simulink model "TESAOffense13"  (R2025b)
settings: Solver=FixedStepAuto  StartTime=0.0  StopTime=SimulationTime  FixedStep=timestep  RelTol=1e-3
values from neighbouring files (symbols this model uses):
  g = 9.81    [TESA_Workspace1.m]
  I = eye(3,3)    [TESA_Workspace1.m]
  K = [1 1 1 1 ... (first row only)    [TESA_Workspace1.m]
  m = 4.34    [TESA_Workspace1.m]    (also in min_snap_Coef.m = length(timepoints) - 1)
settings Model: Creator=worap  LastModifiedBy=btxs
settings DataIOCC: ExternalInput=inputStructure  LoadExternalInput=on

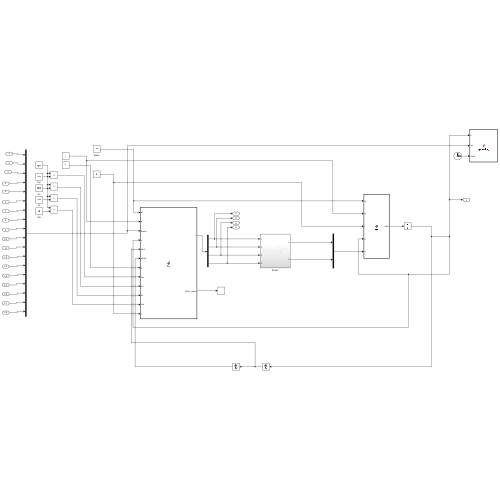
[thumbnail: Simulink's stored preview of the top-level diagram]
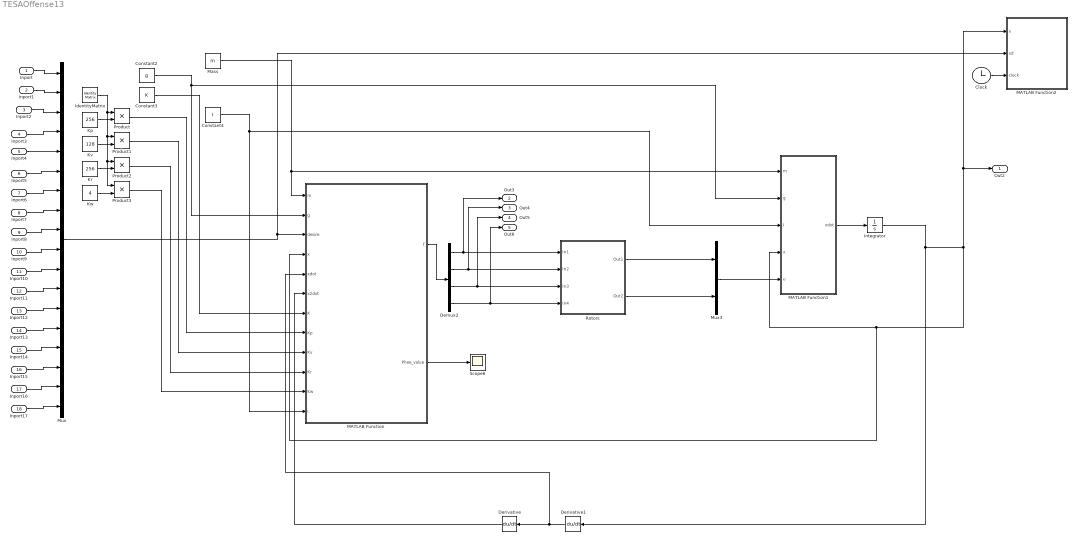
== system TESAOffense13 ==
  Inport : Inport
  Inport1 : Inport  Port=2
  Inport2 : Inport  Port=3
  Inport3 : Inport  Port=4
  Inport4 : Inport  Port=5
  Inport5 : Inport  Port=6
  Inport6 : Inport  Port=7
  Inport7 : Inport  Port=8
  Inport8 : Inport  Port=9
  Inport9 : Inport  Port=10
  Inport10 : Inport  Port=11
  Inport11 : Inport  Port=12
  Inport12 : Inport  Port=13
  Inport13 : Inport  Port=14
  Inport14 : Inport  Port=15
  Inport15 : Inport  Port=16
  Inport16 : Inport  Port=17
  Inport17 : Inport  Port=18
  Clock : Clock
  Constant2 : Constant  Value=g
  Constant3 : Constant  Value=K
  Constant4 : Constant  Value=I
  Demux2 : Demux
  Derivative : Derivative
  Derivative1 : Derivative
  IdentityMatrix : IdentityMatrix  OutputDimensions=3
  Integrator : Integrator  InitialCondition=[0;0;0;0;0;0;1;0;0;0;1;0;0;0;1;0;0;0]
  Kp : Constant  Value=256
  Kr : Constant  Value=256
  Kv : Constant  Value=128
  Kw : Constant  Value=4
  MATLAB Function : MATLAB Function  TreatAsAtomicUnit=on
  MATLAB Function1 : MATLAB Function  TreatAsAtomicUnit=on
  MATLAB Function2 : MATLAB Function  TreatAsAtomicUnit=on
  Mass : Constant  Value=m
  Mux : Mux  Inputs=18
  Mux3 : Mux  Inputs=2
  Product{,1..3} (4 alike) : Product
  Rotors : Subsystem
  Scope6 : Scope
      settings: ActiveDisplayYMinimum=-0.44275151158705367  ActiveDisplayYMaximum=-0.10480685049587157
  Out2 : Outport
  Out3 : Outport  Port=2
  Out4 : Outport  Port=3
  Out5 : Outport  Port=4
  Out6 : Outport  Port=5
  wires:
  Mass/1 -> MATLAB Function1/1(m), MATLAB Function/1(m)
  Demux2/2 -> Out4/1, Rotors/2(In2)
  Rotors/1(Out1) -> Mux3/1
  Rotors/2(Out2) -> Mux3/2
  Demux2/3 -> Out5/1, Rotors/3(In3)
  Demux2/4 -> Out6/1, Rotors/4(In4)
  Constant4/1 -> MATLAB Function1/3(I), MATLAB Function/12(I)
  MATLAB Function/1(f) -> Demux2/1
  Demux2/1 -> Out3/1, Rotors/1(In1)
  Constant2/1 -> MATLAB Function1/2(g), MATLAB Function/2(g)
  Constant3/1 -> MATLAB Function/7(K)
  Product/1 -> MATLAB Function/8(Kp)
  Product1/1 -> MATLAB Function/9(Kv)
  Product3/1 -> MATLAB Function/11(Kw)
  Product2/1 -> MATLAB Function/10(Kr)
  MATLAB Function/2(Phee_value) -> Scope6/1
  Mux3/1 -> MATLAB Function1/5(u)
  MATLAB Function1/1(xdot) -> Integrator/1
  Integrator/1 -> Derivative1/1, MATLAB Function/4(x), MATLAB Function1/4(x), MATLAB Function2/1(x), Out2/1
  Mux/1 -> MATLAB Function2/2(xd), MATLAB Function/3(desire)
  Inport17/1 -> Mux/18
  Inport16/1 -> Mux/17
  Inport15/1 -> Mux/16
  Inport14/1 -> Mux/15
  Inport13/1 -> Mux/14
  Inport12/1 -> Mux/13
  Inport11/1 -> Mux/12
  Inport10/1 -> Mux/11
  Inport9/1 -> Mux/10
  Inport8/1 -> Mux/9
  Inport7/1 -> Mux/8
  Inport6/1 -> Mux/7
  Inport5/1 -> Mux/6
  Inport4/1 -> Mux/5
  Inport3/1 -> Mux/4
  Inport2/1 -> Mux/3
  Inport1/1 -> Mux/2
  Inport/1 -> Mux/1
  Derivative/1 -> MATLAB Function/6(x2dot)
  Derivative1/1 -> MATLAB Function/5(xdot), Derivative/1
  Kp/1 -> Product/2
  IdentityMatrix/1 -> Product3/1, Product2/1, Product1/1, Product/1
  Kv/1 -> Product1/2
  Kr/1 -> Product2/2
  Kw/1 -> Product3/2
  Clock/1 -> MATLAB Function2/3(clock)

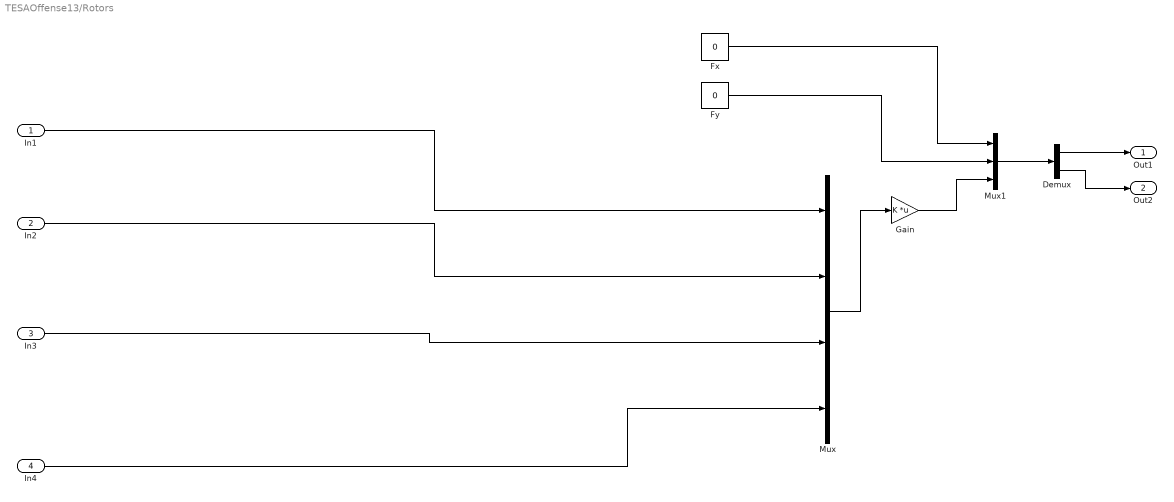
== system TESAOffense13/Rotors ==
  In1 : Inport
  In2 : Inport  Port=2
  In3 : Inport  Port=3
  In4 : Inport  Port=4
  Demux : Demux  Outputs=2
  Fx : Constant  Value=0
  Fy : Constant  Value=0
  Gain : Gain  Gain=K  Multiplication=Matrix(K*u) (u vector)
  Mux : Mux
  Mux1 : Mux  Inputs=3
  Out1 : Outport
  Out2 : Outport  Port=2
  wires:
  Fx/1 -> Mux1/1
  Mux1/1 -> Demux/1
  Fy/1 -> Mux1/2
  Mux/1 -> Gain/1
  Gain/1 -> Mux1/3
  Demux/2 -> Out2/1
  Demux/1 -> Out1/1
  In1/1 -> Mux/1
  In2/1 -> Mux/2
  In3/1 -> Mux/3
  In4/1 -> Mux/4

== matlab function TESAOffense13/MATLAB Function1 ==
  data: m input; g input; I input; x input; u input; xdot output
function xdot = fcn(m,g,I,x,u)

% extract the x-vextor
p = x(1:3,1);
v = x(4:6,1);
R = reshape(x(7:15,1),3,3);
omega = x(16:18,1);

%control signal
f = u(3,1);
M = u(4:6,1);

e3 = [0;0;1];

xdot = zeros(size(x));

xdot(1:3,1) = v;
xdot(4:6,1) = g*e3 - 1/m*f*R*e3;

Rdot = R*hatmap(omega);
xdot(7:15,1) = Rdot(:);
% \ use for optimization
xdot(16:18,1) = I\(M - cross(omega,I*omega));




end

== matlab function TESAOffense13/MATLAB Function ==
  data: m input; g input; f output; Phee_value output; desire input; x input; xdot input; x2dot input; K input; Kp input; Kv input; Kr input; Kw input; I input
function [f,Phee_value]  = fcn(m,g,desire,x,xdot,x2dot,K,Kp,Kv,Kr,Kw,I)

% TODO: implement
xt = desire(1);
yt = desire(2);
zt = desire(3);

dxt = desire(4);
dyt = desire(5);
dzt = desire(6);

ddxt = desire(7);
ddyt = desire(8);
ddzt = desire(9);

dddxt = desire(10);
dddyt = desire(11);
dddzt = desire(12);

ddddxt = desire(13);
ddddyt = desire(14);
ddddzt = desire(15);

psit = desire(16);
dpsit = desire(17);
ddpsit = desire(18);

% constant variable
e3 = [0;0;1];
omega = x(16:18,1);
omegaHat = hatmap(omega);

% r = unit direction vector
rd = [xt;yt;zt];
r = x(1:3,1);

% v = velocity vector
vd = [dxt; dyt; dzt];
v = xdot(1:3,1);

R = reshape(x(7:15,1),3,3);
% ======= find position and velocity error ========
ex = r-rd;
ev = v-vd;

% ======= find rotation desire matrix ========
ddxd = [ddxt; ddyt; ddzt];   

fdes = -(-Kp*ex - Kv*ev - m*g*e3 + m*ddxd);

zbdes = fdes / norm(fdes);    

h = [cos(psit); sin(psit); 0];  
ybdes = cross(zbdes, h);
ybdes = ybdes / norm(ybdes);

xbdes = cross(ybdes, zbdes);

Rdes = [xbdes, ybdes, zbdes];

% ======= find omega desire ========
omegaDes  = [0; 0; dpsit];
dOmegaDes = [0; 0; ddpsit];

% ======= find rotation matrix and omega error ========
er = 0.5 * veemap(Rdes'*R - R'*Rdes);
ew = omega - R'*Rdes*omegaDes;

% ======= find rotor dynamics ========
fz = dot(fdes,R*e3);
M = -(Kr*er)-(Kw*ew)+cross(omega,(I*omega))-(I*((omegaHat*R'*Rdes*omegaDes)-(R'*Rdes*dOmegaDes)));
u = [fz;M];

f = K \ u;

Phee_value = 0.5 * trace( I - (Rdes') * R );
end

== matlab function TESAOffense13/MATLAB Function2 ==
  data: x input; xd input; clock input
function api_calling(x, xd, clock)

coder.extrinsic('weboptions', 'webwrite', 'datetime');

% Prepare payload for API
url = 'http://localhost:3000/drone-location';
% url = 'http://192.168.10.181/api/v1/attacks-accuracy';
lat_init = 14.303128109956759;
long_init = 1.011545747324440e+02;
alt_init = 38;

% Convert from NED to LLA
realPosition = ned2lla(x(1:3,1)', [lat_init long_init alt_init], "ellipsoid");
desirePosition = ned2lla(xd(1:3,1)', [lat_init long_init alt_init], "ellipsoid");

% Compute speed (magnitude of velocity vector)
realSpeed = norm(x(4:6,1)); 

payload = struct();
payload.droneId = 101;
payload.realLat = realPosition(1,1);
payload.realLong = realPosition(1,2);
payload.realAlt = realPosition(1,3);
payload.desireLat = desirePosition(1,1);
payload.desireLong = desirePosition(1,2);
payload.desireAlt = desirePosition(1,3);
payload.speed = realSpeed;
payload.timeRange = 20;
payload.currentTime = clock;
payload.meanAccuracy = NaN;

options = weboptions('MediaType', 'application/json');
webwrite(url, payload, options);

end
